simulink model "module"  (R2020b)
settings: Solver=VariableStepAuto  StartTime=0.0  StopTime=t_end  RelTol=1e-6
values from neighbouring files (symbols this model uses):
  R_ext = 0.002    [main.m]    (also in main_cell.m = 0.0066)
undefined symbols (not defined in the file or in its folder): cells
libraries: nesl_utility x16, fl_lib x7, LiBatteryElements_lib x3, simulink x1
settings Model: Creator=Vivian  LastModifiedBy=Vivian
settings SolverCC: ZeroCrossAlgorithm=Adaptive

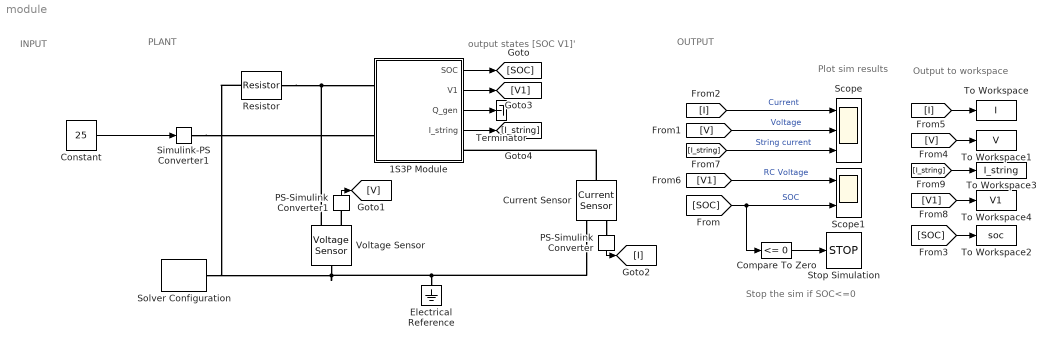
== system module ==
  note: output states [SOC V1]'
  note: Output to workspace
  note: Plot sim results
  note: Stop the sim if SOC<=0
  note: PLANT
  note: INPUT
  note: OUTPUT
  1S3P Module : Subsystem
  Compare To Zero : simulink/Logic and Bit Operations/Compare To Zero  relop=<=  OutDataTypeStr=boolean
  Constant : Constant  Value=25
  Current Sensor : fl_lib/Electrical/Electrical Sensors/Current Sensor
  Electrical Reference : fl_lib/Electrical/Electrical Elements/Electrical Reference
  PS-Simulink Converter : nesl_utility/PS-Simulink Converter  PhysicalDomain=network_engine_domain  SubClassName=ps_output  LeftPortType=input  RightPortType=output  PseudoPeriodic=off  Frequencies=[]  Unit=inherit  AffineConversion=off
  PS-Simulink Converter1 : nesl_utility/PS-Simulink Converter  PhysicalDomain=network_engine_domain  SubClassName=ps_output  LeftPortType=input  RightPortType=output  PseudoPeriodic=off  Frequencies=[]  Unit=inherit  AffineConversion=off
  Resistor : fl_lib/Electrical/Electrical Elements/Resistor  R=R_ext Ohm  i_specify=off  i_priority=None  i=0 A  i_nominal_specify=off  i_nominal_unit=A  i_nominal_value=1  v_specify=off  v_priority=None  v=0 V  v_nominal_specify=off  v_nominal_unit=V  v_nominal_value=1
  Scope : Scope  NumInputPorts=3
  Scope1 : Scope  NumInputPorts=2
  Simulink-PS Converter1 : nesl_utility/Simulink-PS Converter  PhysicalDomain=network_engine_domain  SubClassName=ps_input  LeftPortType=input  RightPortType=output  PseudoPeriodic=off  Frequencies=[]  NoiseDistribution=none  NoiseParameters=[]  Unit=1  AffineConversion=off  FilteringAndDerivatives=provide  SimscapeFilterOrder=1  InputFilterTimeConstant=0.001  UdotUserProvided=0
  Solver Configuration : nesl_utility/Solver Configuration  PhysicalDomain=network_engine_domain  SubClassName=solver  LeftPortType=input  RightPortType=generic  Tones=[]  Harmonics=[]  SimulateNoise=off  Profile=off  UseLocalSampling=off  EnableSwitchedLinearOptims=on  FrequencyDomain=off  UseCCode=off  RelTol=0.001  AbsTol=1e-06  MinStep=1e-09  ToWorkspace=off  RevertToSquareIcSolve=off  NumHomotopyIterations=100  PhasorMode=off  PhasorModeNumHarmonics=1  DoDC=off  ResidualTolerance=1e-09  UseLocalSolver=off  LocalSolverChoice=NE_BACKWARD_EULER_ADVANCER  LocalSolverSampleTime=0.001  DoFixedCost=off  MaxNonlinIter=3  MaxModeIter=2  ComputeImpulses=off  ImpulseIterations=2  LinearAlgebra=auto  EquationFormulation=NE_TIME_EF  DelaysMemoryBudget=1024  AutomaticFiltering=on  FilteringTimeConstant=0.001  PartitionStorageMethod=AS_NEEDED  PartitionMemoryBudget=1024  PartitionMethod=ROBUST
  Stop Simulation : Stop
  Terminator : Terminator
  To Workspace : ToWorkspace  VariableName=I  SaveFormat=Timeseries  SampleTime=-1
  To Workspace1 : ToWorkspace  VariableName=V  SaveFormat=Timeseries  SampleTime=-1
  To Workspace2 : ToWorkspace  VariableName=soc  SaveFormat=Timeseries  SampleTime=-1
  To Workspace3 : ToWorkspace  VariableName=I_string  SaveFormat=Timeseries  SampleTime=-1
  To Workspace4 : ToWorkspace  VariableName=V1  SaveFormat=Timeseries  SampleTime=-1
  Voltage Sensor : fl_lib/Electrical/Electrical Sensors/Voltage Sensor
  wires:
  Compare To Zero/1 -> Stop Simulation/1
  1S3P Module/1(SOC) -> [SOC]
  [SOC] -> Compare To Zero/1, Scope1/2  "SOC"
  [V] -> Scope/2  "Voltage"
  PS-Simulink Converter/1 -> [I]
  PS-Simulink Converter1/1 -> [V]
  [I] -> Scope/1  "Current"
  [I] -> To Workspace/1
  [V] -> To Workspace1/1
  [SOC] -> To Workspace2/1
  Constant/1 -> Simulink-PS Converter1/1
  1S3P Module/3(Q_gen) -> Terminator/1
  1S3P Module/2(V1) -> [V1]
  1S3P Module/4(I_string) -> [I_string]
  [I_string] -> Scope/3  "String current"
  [V1] -> To Workspace4/1
  [I_string] -> To Workspace3/1
  [V1] -> Scope1/1  "RC Voltage"
  connections:
  Current Sensor/RConn2 -- Electrical Reference/LConn1 -- Resistor/LConn1 -- Solver Configuration/RConn1 -- Voltage Sensor/LConn1
  Voltage Sensor/RConn1 -- PS-Simulink Converter1/LConn1
  Voltage Sensor/RConn2 -- Resistor/RConn1 -- 1S3P Module/LConn1
  Current Sensor/LConn1 -- 1S3P Module/RConn1
  Current Sensor/RConn1 -- PS-Simulink Converter/LConn1
  Simulink-PS Converter1/RConn1 -- 1S3P Module/LConn2

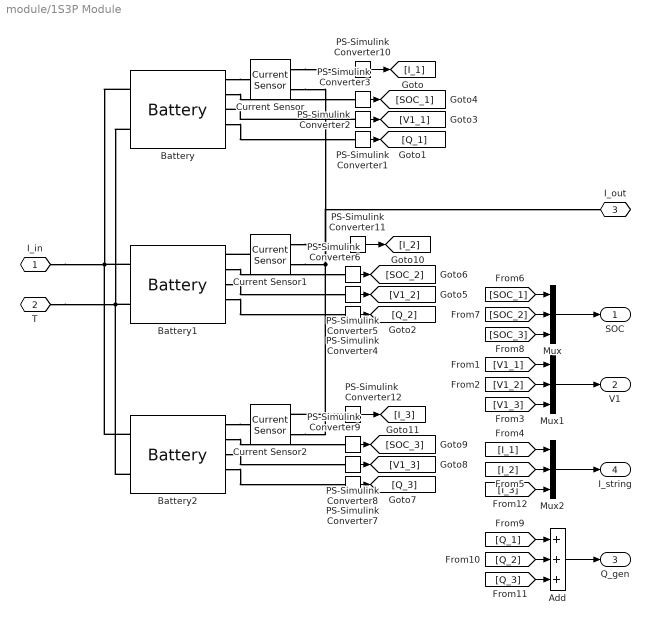
== system module/1S3P Module ==
  Add : Sum  Inputs=+++
  Battery : LiBatteryElements_lib/Battery  OCV=cells(1).OCV  Em_Table_unit=V  SOC_OCV=cells(1).SOC_OCV  capacity=cells(1).capacity  SOC_0=cells(1).SOC_0  Rs=cells(1).Rs  Rs_Table_unit=Ohm  SOC_RC_Rs=cells(1).SOC_RC  T_RC_Rs=cells(1).T_RC  Temp_Table_unit_Rs=degC  R1=cells(1).R1  R1_Table_unit_copy=Ohm  SOC_RC_R1=cells(1).SOC_RC  T_RC_R1=cells(1).T_RC  Temp_Table_unit_R1=degC  C1=cells(1).C1  C1_Table_unit=F  SOC_RC_C1=cells(1).SOC_RC  T_RC_C1=cells(1).T_RC  Temp_Table_unit_C1=degC  v0=0 V
      settings: SourceProductBaseCode=SS
  Battery1 : LiBatteryElements_lib/Battery  OCV=cells(2).OCV  Em_Table_unit=V  SOC_OCV=cells(2).SOC_OCV  capacity=cells(2).capacity  SOC_0=cells(2).SOC_0  Rs=cells(2).Rs  Rs_Table_unit=Ohm  SOC_RC_Rs=cells(2).SOC_RC  T_RC_Rs=cells(2).T_RC  Temp_Table_unit_Rs=degC  R1=cells(2).R1  R1_Table_unit_copy=Ohm  SOC_RC_R1=cells(2).SOC_RC  T_RC_R1=cells(2).T_RC  Temp_Table_unit_R1=degC  C1=cells(2).C1  C1_Table_unit=F  SOC_RC_C1=cells(2).SOC_RC  T_RC_C1=cells(2).T_RC  Temp_Table_unit_C1=degC  v0=0 V
      settings: SourceProductBaseCode=SS
  Battery2 : LiBatteryElements_lib/Battery  OCV=cells(3).OCV  Em_Table_unit=V  SOC_OCV=cells(3).SOC_OCV  capacity=cells(3).capacity  SOC_0=cells(3).SOC_0  Rs=cells(3).Rs  Rs_Table_unit=Ohm  SOC_RC_Rs=cells(3).SOC_RC  T_RC_Rs=cells(3).T_RC  Temp_Table_unit_Rs=degC  R1=cells(3).R1  R1_Table_unit_copy=Ohm  SOC_RC_R1=cells(3).SOC_RC  T_RC_R1=cells(3).T_RC  Temp_Table_unit_R1=degC  C1=cells(3).C1  C1_Table_unit=F  SOC_RC_C1=cells(3).SOC_RC  T_RC_C1=cells(3).T_RC  Temp_Table_unit_C1=degC  v0=0 V
      settings: SourceProductBaseCode=SS
  Current Sensor : fl_lib/Electrical/Electrical Sensors/Current Sensor
  Current Sensor1 : fl_lib/Electrical/Electrical Sensors/Current Sensor
  Current Sensor2 : fl_lib/Electrical/Electrical Sensors/Current Sensor
  Mux : Mux  Inputs=3
  Mux1 : Mux  Inputs=3
  Mux2 : Mux  Inputs=3
  PS-Simulink Converter{1..12} (12 alike) : nesl_utility/PS-Simulink Converter  PhysicalDomain=network_engine_domain  SubClassName=ps_output  LeftPortType=input  RightPortType=output  PseudoPeriodic=off  Frequencies=[]  Unit=inherit  AffineConversion=off
  I_in : PMIOPort  Side=Left
  T : PMIOPort  Port=2  Side=Left
  I_out : PMIOPort  Port=3  Side=Right
  SOC : Outport
  V1 : Outport  Port=2
  Q_gen : Outport  Port=3
  I_string : Outport  Port=4
  wires:
  [SOC_3] -> Mux/3
  [SOC_1] -> Mux/1
  [SOC_2] -> Mux/2
  [Q_2] -> Add/2
  [Q_1] -> Add/1
  Mux/1 -> SOC/1
  [Q_3] -> Add/3
  PS-Simulink Converter2/1 -> [V1_1]
  PS-Simulink Converter3/1 -> [SOC_1]
  Add/1 -> Q_gen/1
  PS-Simulink Converter1/1 -> [Q_1]
  PS-Simulink Converter4/1 -> [Q_2]
  PS-Simulink Converter5/1 -> [V1_2]
  PS-Simulink Converter6/1 -> [SOC_2]
  PS-Simulink Converter7/1 -> [Q_3]
  PS-Simulink Converter8/1 -> [V1_3]
  PS-Simulink Converter9/1 -> [SOC_3]
  Mux1/1 -> V1/1
  [V1_2] -> Mux1/2
  [V1_1] -> Mux1/1
  [V1_3] -> Mux1/3
  PS-Simulink Converter10/1 -> [I_1]
  PS-Simulink Converter11/1 -> [I_2]
  PS-Simulink Converter12/1 -> [I_3]
  [I_2] -> Mux2/2
  Mux2/1 -> I_string/1
  [I_3] -> Mux2/3
  [I_1] -> Mux2/1
  connections:
  Battery/RConn2 -- PS-Simulink Converter3/LConn1
  Current Sensor2/RConn2 -- I_out/RConn1 -- Current Sensor/RConn2 -- Current Sensor1/RConn2
  I_in/RConn1 -- Battery2/LConn1 -- Battery/LConn1 -- Battery1/LConn1
  PS-Simulink Converter2/LConn1 -- Battery/RConn3
  T/RConn1 -- Battery2/LConn2 -- Battery1/LConn2 -- Battery/LConn2
  Battery/RConn4 -- PS-Simulink Converter1/LConn1
  Battery1/RConn2 -- PS-Simulink Converter6/LConn1
  Battery1/RConn3 -- PS-Simulink Converter5/LConn1
  Battery1/RConn4 -- PS-Simulink Converter4/LConn1
  Battery2/RConn2 -- PS-Simulink Converter9/LConn1
  Battery2/RConn3 -- PS-Simulink Converter8/LConn1
  Battery2/RConn4 -- PS-Simulink Converter7/LConn1
  Current Sensor/RConn1 -- PS-Simulink Converter10/LConn1
  Current Sensor1/RConn1 -- PS-Simulink Converter11/LConn1
  PS-Simulink Converter12/LConn1 -- Current Sensor2/RConn1
  Battery2/RConn1 -- Current Sensor2/LConn1
  Current Sensor1/LConn1 -- Battery1/RConn1
  Battery/RConn1 -- Current Sensor/LConn1
